simulink model "goldenSectionMethod_th"  (R2018b)
settings: Solver=VariableStepAuto  StartTime=0.0  StopTime=10.0  RelTol=1e-3
libraries: courseFollow_cl x1
settings Model: Creator=James Reed  LastModifiedBy=James Reed

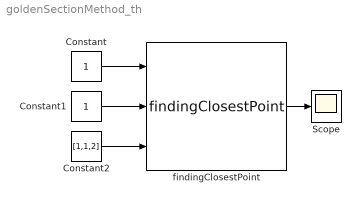
== system goldenSectionMethod_th ==
  Constant : Constant
  Constant1 : Constant
  Constant2 : Constant  Value=[1,1,2]
  Scope : Scope
  findingClosestPoint : courseFollow_cl/courseFollow/findingClosestPoint  SystemSampleTime=-1
  wires:
  Constant/1 -> findingClosestPoint/1
  Constant1/1 -> findingClosestPoint/2
  Constant2/1 -> findingClosestPoint/3
  findingClosestPoint/1 -> Scope/1
